simulink model "winter_simulink_with_PC_generator_control_EKF"  (R2022a)
settings: Solver=FixedStepAuto  StartTime=0  StopTime=50  FixedStep=simulation.time_step_H
values from neighbouring files (symbols this model uses):
  B_eq = param{6}    [measurement_2states.m]    (also in measurement_2states_3mes.m; measurement_3measure.m)
  rho = param{2}    [measurement_3measure.m]
undefined symbols (not defined in the file or in its folder): blade, Gc, gearbox, generator, generator_kd, generator_ki, generator_kp, generator_tau_d1, I_eq, IMM, lambda_vector, lookup_cP, omega_R, omega_rated, omega_rated_GE, pitch_range, pitch_vector, R_TG, rotor, simulation, T_R0, wind
settings Model: Creator=Niccolò  LastModifiedBy=Niccolò
settings SolverCC: ZeroCrossAlgorithm=Adaptive
settings DebuggingCC: IgnoredZcDiagnostic=none

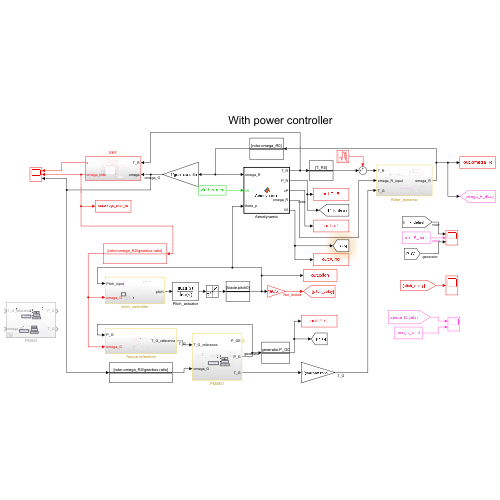
[thumbnail: Simulink's stored preview of the top-level diagram]
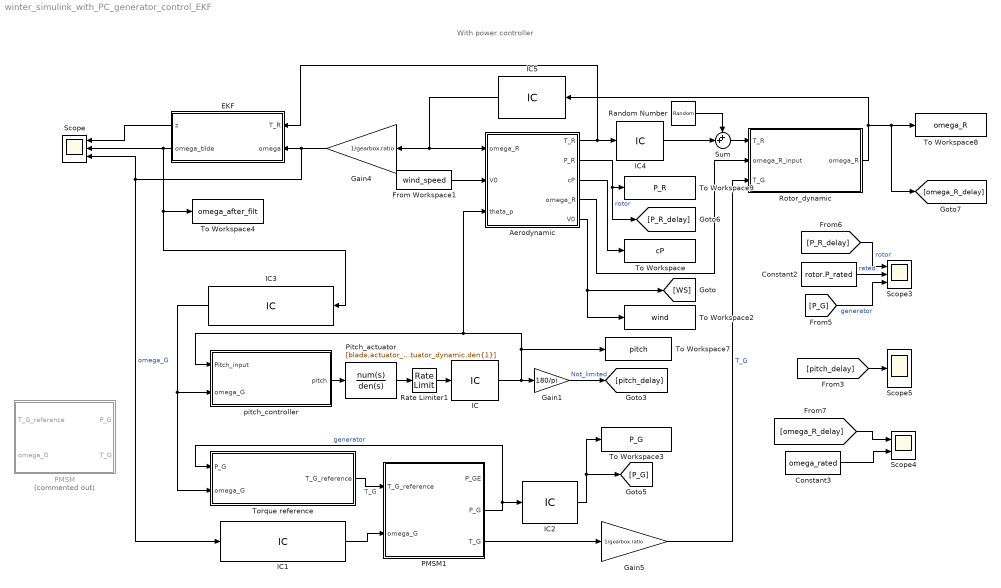
== system winter_simulink_with_PC_generator_control_EKF ==
  note: With power controller
  Aerodynamic : MATLAB Function  TreatAsAtomicUnit=on
  Constant2 : Constant  Value=rotor.P_rated
  Constant3 : Constant  Value=omega_rated
  EKF : Subsystem
  From Workspace1 : FromWorkspace  VariableName=wind_speed  SampleTime=1/wind.sample_f
  Gain1 : Gain  Gain=180/pi  SampleTime=simulation.time_step_H
  Gain4 : Gain  Gain=1/gearbox.ratio
  Gain5 : Gain  Gain=1/gearbox.ratio
  IC : InitialCondition  Value=blade.pitch0
  IC1 : InitialCondition  Value=rotor.omega_R0/gearbox.ratio
  IC2 : InitialCondition  Value=generator.P_G0
  IC3 : InitialCondition  Value=rotor.omega_R0/gearbox.ratio
  IC4 : InitialCondition  Value=T_R0
  IC5 : InitialCondition  Value=rotor.omega_R0
  PMSM : Subsystem  Commented=on
  PMSM1 : Subsystem
  Pitch_actuator : TransferFcn  Numerator=[blade.actuator_dynamic.num{1}]  Denominator=[blade.actuator_dynamic.den{1}]
  Random Number : RandomNumber  Variance=IMM.Q  SampleTime=simulation.time_step_H
  Rate Limiter1 : RateLimiter  RisingSlewLimit=blade.pitch_rate  FallingSlewLimit=-blade.pitch_rate  SampleTimeMode=inherited
  Rotor_dynamic : Subsystem
  Scope : Scope  NumInputPorts=3
  Scope3 : Scope  NumInputPorts=3
  Scope4 : Scope  NumInputPorts=2
  Scope5 : Scope
  Sum : Sum  Inputs=++|
  To Workspace : ToWorkspace  VariableName=cP  SaveFormat=Timeseries  SampleTime=-1
  To Workspace2 : ToWorkspace  VariableName=wind  SaveFormat=Timeseries  SampleTime=-1
  To Workspace3 : ToWorkspace  VariableName=P_G  SaveFormat=Timeseries  SampleTime=-1
  To Workspace4 : ToWorkspace  VariableName=omega_after_filt  SaveFormat=Timeseries  SampleTime=-1
  To Workspace7 : ToWorkspace  VariableName=pitch  SaveFormat=Timeseries  SampleTime=-1
  To Workspace8 : ToWorkspace  VariableName=omega_R  SaveFormat=Timeseries  SampleTime=-1
  To Workspace9 : ToWorkspace  VariableName=P_R  SaveFormat=Timeseries  SampleTime=-1
  Torque reference : Subsystem
  pitch_controller : Subsystem
  wires:
  From Workspace1/1 -> Aerodynamic/2("V0 ")
  Aerodynamic/2(P_R) -> [P_R_delay], To Workspace9/1  "rotor"
  [pitch_delay] -> Scope5/1
  Gain4/1 -> EKF/2(omega), IC1/1, Scope/3  "omega_G"
  Rate Limiter1/1 -> IC/1
  [P_R_delay] -> Scope3/1  "rotor"
  Constant3/1 -> Scope4/2
  Constant2/1 -> Scope3/2  "rated"
  [omega_R_delay] -> Scope4/1
  Gain1/1 -> [pitch_delay]  "Not_limited"
  Aerodynamic/1(T_R) -> EKF/1(T_R), IC4/1
  [P_G] -> Scope3/3  "generator"
  pitch_controller/1(pitch) -> Pitch_actuator/1
  Pitch_actuator/1 -> Rate Limiter1/1
  Gain5/1 -> Rotor_dynamic/3(T_G)  "T_G"
  IC/1 -> To Workspace7/1, Aerodynamic/3(theta_p), pitch_controller/1(Pitch_input), Gain1/1
  IC3/1 -> pitch_controller/2(omega_G), Torque reference/2(omega_G)
  IC2/1 -> To Workspace3/1, [P_G]
  IC4/1 -> Sum/2
  Rotor_dynamic/1(omega_R) -> IC5/1, [omega_R_delay], To Workspace8/1
  IC5/1 -> Aerodynamic/1("omega_R "), Gain4/1
  Aerodynamic/3(cP) -> To Workspace/1
  EKF/2(omega_tilde) -> To Workspace4/1, IC3/1, Scope/2
  Aerodynamic/4(omega_R) -> Rotor_dynamic/2(omega_R_input)
  Aerodynamic/5(V0) -> To Workspace2/1, [WS]
  PMSM1/2(P_G) -> Torque reference/1(P_G), IC2/1  "generator"
  IC1/1 -> PMSM1/2(omega_G)
  Torque reference/1(T_G_reference) -> PMSM1/1(T_G_reference)  "T_G"
  PMSM1/3(T_G) -> Gain5/1
  EKF/1(z) -> Scope/1
  Sum/1 -> Rotor_dynamic/1(T_R)
  Random Number/1 -> Sum/1

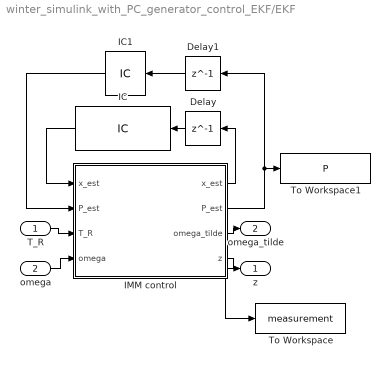
== system winter_simulink_with_PC_generator_control_EKF/EKF ==
  T_R : Inport
  omega : Inport  Port=2
  Delay : Delay  DelayLength=1
  Delay1 : Delay  DelayLength=1
  IC : InitialCondition  Value=rotor.omega_R0
  IC1 : InitialCondition  Value=1e2
  IMM control : MATLAB Function  TreatAsAtomicUnit=on
  To Workspace : ToWorkspace  VariableName=measurement  SaveFormat=Timeseries  SampleTime=-1
  To Workspace1 : ToWorkspace  VariableName=P  SaveFormat=Timeseries  SampleTime=-1
  z : Outport
  omega_tilde : Outport  Port=2
  wires:
  IMM control/3(omega_tilde) -> omega_tilde/1
  Delay1/1 -> IC1/1
  IMM control/1(x_est) -> Delay/1
  Delay/1 -> IC/1
  IMM control/2(P_est) -> Delay1/1, To Workspace1/1
  T_R/1 -> IMM control/3(T_R)
  omega/1 -> IMM control/4(omega)
  IC1/1 -> IMM control/2("P_est ")
  IC/1 -> IMM control/1("x_est ")
  IMM control/4(z) -> To Workspace/1, z/1

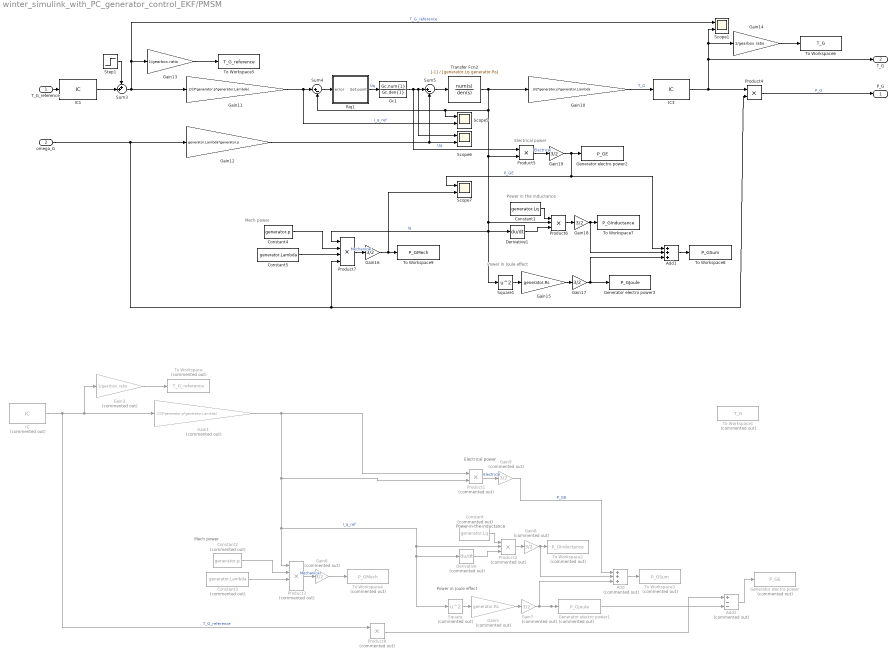
== system winter_simulink_with_PC_generator_control_EKF/PMSM ==
  note: Power in Joule effect
  note: Power in the inductance
  note: Electrical power
  note: Mech power
  note: Power in the inductance
  note: Electrical power
  note: Mech power
  note: Power in Joule effect
  T_G_reference : Inport
  omega_G : Inport  Port=2
  Add : Sum  Commented=on  Inputs=3
  Add1 : Sum  Inputs=3
  Add2 : Sum  Commented=on  Inputs=+--
  Constant : Constant  Commented=on  Value=generator.Lq
  Constant1 : Constant  Value=generator.Lq
  Constant2 : Constant  Commented=on  Value=generator.p
  Constant3 : Constant  Commented=on  Value=generator.Lambda
  Constant4 : Constant  Value=generator.p
  Constant5 : Constant  Value=generator.Lambda
  Derivative : Derivative  Commented=on
  Derivative1 : Derivative
  Gain1 : Gain  Commented=on  Gain=2/(3*generator.p*generator.Lambda)
  Gain10 : Gain  Gain=3/2*generator.p*generator.Lambda
  Gain11 : Gain  Gain=2/(3*generator.p*generator.Lambda)
  Gain12 : Gain  Gain=generator.Lambda*generator.p
  Gain13 : Gain  Gain=1/gearbox.ratio
  Gain14 : Gain  Gain=1/gearbox.ratio
  Gain15 : Gain  Gain=generator.Rs
  Gain{16..19} (4 alike) : Gain  Gain=3/2
  Gain3 : Gain  Commented=on  Gain=1/gearbox.ratio
  Gain5 : Gain  Commented=on  Gain=generator.Rs
  Gain{6..9} (4 alike) : Gain  Commented=on  Gain=3/2
  Gc1 : TransferFcn  Numerator=Gc.num{1}  Denominator=Gc.den{1}
  Generator electro power : ToWorkspace  Commented=on  VariableName=P_GE  SaveFormat=Timeseries  SampleTime=-1
  Generator electro power1 : ToWorkspace  Commented=on  VariableName=P_GJoule  SaveFormat=Timeseries  SampleTime=-1
  Generator electro power2 : ToWorkspace  VariableName=P_GE  SaveFormat=Timeseries  SampleTime=-1
  Generator electro power3 : ToWorkspace  VariableName=P_GJoule  SaveFormat=Timeseries  SampleTime=-1
  IC : InitialCondition  Commented=on  Value=generator.T_G0
  IC1 : InitialCondition  Value=generator.T_G0
  IC3 : InitialCondition  Value=generator.T_G0
  Product1 : Product  Commented=on
  Product2 : Product  Commented=on  Inputs=3
  Product3 : Product  Commented=on  Inputs=4
  Product4 : Product
  Product5 : Product
  Product6 : Product  Inputs=3
  Product7 : Product  Inputs=4
  Product8 : Product  Commented=on
  Riq1 : Subsystem
  Scope{1,5..7} (4 alike) : Scope  NumInputPorts=2
  Square : Math  Commented=on  Operator=square
  Square1 : Math  Operator=square
  Step1 : Step  Time=0.5  SampleTime=0
  Sum3 : Sum  Inputs=++|
  Sum4 : Sum  Inputs=|+-
  Sum5 : Sum  Inputs=|+-
  To Workspace : ToWorkspace  Commented=on  VariableName=T_G_reference  SaveFormat=Timeseries  SampleTime=-1
  To Workspace1 : ToWorkspace  Commented=on  VariableName=T_G  SaveFormat=Timeseries  SampleTime=-1
  To Workspace2 : ToWorkspace  Commented=on  VariableName=P_GInductance  SaveFormat=Timeseries  SampleTime=-1
  To Workspace3 : ToWorkspace  Commented=on  VariableName=P_GSum  SaveFormat=Timeseries  SampleTime=-1
  To Workspace4 : ToWorkspace  Commented=on  VariableName=P_GMech  SaveFormat=Timeseries  SampleTime=-1
  To Workspace5 : ToWorkspace  VariableName=T_G_reference  SaveFormat=Timeseries  SampleTime=-1
  To Workspace6 : ToWorkspace  VariableName=T_G  SaveFormat=Timeseries  SampleTime=-1
  To Workspace7 : ToWorkspace  VariableName=P_GInductance  SaveFormat=Timeseries  SampleTime=-1
  To Workspace8 : ToWorkspace  VariableName=P_GSum  SaveFormat=Timeseries  SampleTime=-1
  To Workspace9 : ToWorkspace  VariableName=P_GMech  SaveFormat=Timeseries  SampleTime=-1
  Transfer Fcn2 : TransferFcn  Numerator=[-1]  Denominator=[generator.Lq generator.Rs]
  P_G : Outport
  T_G : Outport  Port=2
  wires:
  Gain1/1 -> Product1/1, Square/1, Derivative/1, Product2/2, Product3/1, Product1/2  "I_q_ref"
  IC/1 -> Product8/1, Gain1/1, Gain3/1  "T_G_reference"
  Gain3/1 -> To Workspace/1
  Gain5/1 -> Gain7/1
  Square/1 -> Gain5/1
  Derivative/1 -> Product2/3
  Constant/1 -> Product2/1
  Product2/1 -> Gain8/1
  Add/1 -> To Workspace3/1
  Constant2/1 -> Product3/2
  Constant3/1 -> Product3/3
  Product3/1 -> Gain6/1  "Mechanical"
  Product1/1 -> Gain9/1  "Electrical"
  Gain6/1 -> To Workspace4/1
  Gain7/1 -> Add2/3, Generator electro power1/1, Add/3
  Gain8/1 -> Add/2, To Workspace2/1
  Gain9/1 -> Add/1  "P_GE"
  IC1/1 -> Sum3/2
  Product4/1 -> P_G/1  "P_G"
  Gain14/1 -> To Workspace6/1
  Gain19/1 -> Add1/1, Scope7/1, Generator electro power2/1  "P_GE"
  IC3/1 -> Product4/1, T_G/1, Scope1/2, Gain14/1
  Add1/1 -> To Workspace8/1
  Gain12/1 -> Scope6/2, Sum5/2
  Gain16/1 -> Scope7/2, To Workspace9/1
  Constant4/1 -> Product7/2
  omega_G/1 -> Product4/2, Product7/4, Gain12/1
  Square1/1 -> Gain15/1
  Constant5/1 -> Product7/3
  Product7/1 -> Gain16/1  "Mechanical"
  Derivative1/1 -> Product6/3
  Gain15/1 -> Gain17/1
  Constant1/1 -> Product6/1
  Product5/1 -> Gain19/1  "Electrical"
  Product6/1 -> Gain18/1
  Riq1/1(Set point) -> Gc1/1  "Uq"
  Gain11/1 -> Scope5/2, Sum4/1  "I_q_ref"
  Sum4/1 -> Riq1/1(error)
  Gain13/1 -> To Workspace5/1
  Step1/1 -> Sum3/1
  Gain10/1 -> IC3/1  "T_G"
  Sum3/1 -> Gain11/1, Scope1/1, Gain13/1  "T_G_reference"
  Transfer Fcn2/1 -> Gain10/1, Scope5/1, Sum4/2, Product5/2, Product7/1, Square1/1, Derivative1/1, Product6/2  "Iq"
  Sum5/1 -> Transfer Fcn2/1
  Gain18/1 -> To Workspace7/1, Add1/2
  Gain17/1 -> Generator electro power3/1, Add1/3
  Product8/1 -> Add2/1
  Add2/1 -> Generator electro power/1
  T_G_reference/1 -> IC1/1
  Gc1/1 -> Product5/1, Scope6/1, Sum5/1  "Uq"

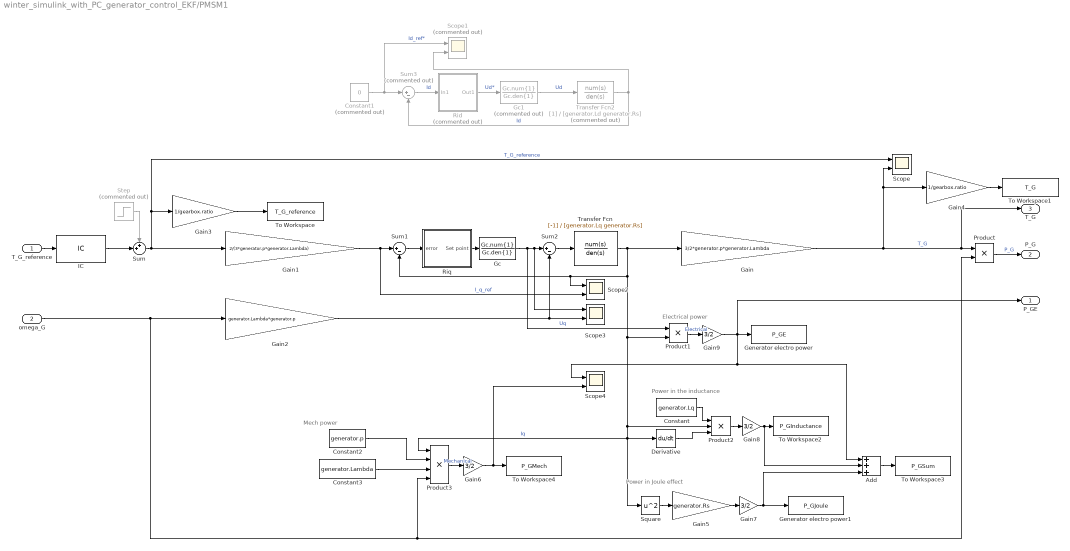
== system winter_simulink_with_PC_generator_control_EKF/PMSM1 ==
  note: Power in Joule effect
  note: Power in the inductance
  note: Electrical power
  note: Mech power
  T_G_reference : Inport
  omega_G : Inport  Port=2
  Add : Sum  Inputs=3
  Constant : Constant  Value=generator.Lq
  Constant1 : Constant  Commented=on  Value=0
  Constant2 : Constant  Value=generator.p
  Constant3 : Constant  Value=generator.Lambda
  Derivative : Derivative
  Gain : Gain  Gain=3/2*generator.p*generator.Lambda
  Gain1 : Gain  Gain=2/(3*generator.p*generator.Lambda)
  Gain2 : Gain  Gain=generator.Lambda*generator.p
  Gain3 : Gain  Gain=1/gearbox.ratio
  Gain4 : Gain  Gain=1/gearbox.ratio
  Gain5 : Gain  Gain=generator.Rs
  Gain{6..9} (4 alike) : Gain  Gain=3/2
  Gc : TransferFcn  Numerator=Gc.num{1}  Denominator=Gc.den{1}
  Gc1 : TransferFcn  Commented=on  Numerator=Gc.num{1}  Denominator=Gc.den{1}
  Generator electro power : ToWorkspace  VariableName=P_GE  SaveFormat=Timeseries  SampleTime=-1
  Generator electro power1 : ToWorkspace  VariableName=P_GJoule  SaveFormat=Timeseries  SampleTime=-1
  IC : InitialCondition  Value=generator.T_G0
  Product : Product
  Product1 : Product
  Product2 : Product  Inputs=3
  Product3 : Product  Inputs=4
  Rid : Subsystem  Commented=on
  Riq : Subsystem
  Scope{,2..4} (4 alike) : Scope  NumInputPorts=2
  Scope1 : Scope  Commented=on  NumInputPorts=2
  Square : Math  Operator=square
  Step : Step  Commented=on  Time=0.5  SampleTime=0
  Sum : Sum  Inputs=++|
  Sum1 : Sum  Inputs=|+-
  Sum2 : Sum  Inputs=|+-
  Sum3 : Sum  Commented=on  Inputs=|+-
  To Workspace : ToWorkspace  VariableName=T_G_reference  SaveFormat=Timeseries  SampleTime=-1
  To Workspace1 : ToWorkspace  VariableName=T_G  SaveFormat=Timeseries  SampleTime=-1
  To Workspace2 : ToWorkspace  VariableName=P_GInductance  SaveFormat=Timeseries  SampleTime=-1
  To Workspace3 : ToWorkspace  VariableName=P_GSum  SaveFormat=Timeseries  SampleTime=-1
  To Workspace4 : ToWorkspace  VariableName=P_GMech  SaveFormat=Timeseries  SampleTime=-1
  Transfer Fcn : TransferFcn  Numerator=[-1]  Denominator=[generator.Lq generator.Rs]
  Transfer Fcn2 : TransferFcn  Commented=on  Denominator=[generator.Ld generator.Rs]
  P_GE : Outport
  P_G : Outport  Port=2
  T_G : Outport  Port=3
  wires:
  Gc/1 -> Product1/1, Scope3/1, Sum2/1  "Uq"
  Gain/1 -> T_G/1, Product/1, Gain4/1, Scope/2  "T_G"
  Riq/1(Set point) -> Gc/1
  Sum1/1 -> Riq/1(error)
  Transfer Fcn/1 -> Gain/1, Scope2/1, Sum1/2, Product1/2, Product3/1, Square/1, Derivative/1, Product2/2  "Iq"
  Product/1 -> P_G/1  "P_G"
  Gain1/1 -> Scope2/2, Sum1/1  "I_q_ref"
  Sum/1 -> Gain1/1, Scope/1, Gain3/1  "T_G_reference"
  T_G_reference/1 -> IC/1
  Step/1 -> Sum/1
  Sum2/1 -> Transfer Fcn/1
  Gain3/1 -> To Workspace/1
  IC/1 -> Sum/2
  Gain5/1 -> Gain7/1
  Square/1 -> Gain5/1
  Derivative/1 -> Product2/3
  Constant/1 -> Product2/1
  Product2/1 -> Gain8/1
  Gc1/1 -> Transfer Fcn2/1  "Ud"
  Rid/1(Out1) -> Gc1/1  "Ud*"
  Transfer Fcn2/1 -> Sum3/2, Scope1/2  "Id"
  Constant1/1 -> Scope1/1, Sum3/1  "Id_ref*"
  Sum3/1 -> Rid/1(In1)  "Id"
  Add/1 -> To Workspace3/1
  Constant2/1 -> Product3/2
  Constant3/1 -> Product3/3
  Product3/1 -> Gain6/1  "Mechanical"
  Product1/1 -> Gain9/1  "Electrical"
  Gain2/1 -> Scope3/2, Sum2/2
  omega_G/1 -> Product/2, Product3/4, Gain2/1
  Gain6/1 -> Scope4/2, To Workspace4/1
  Gain7/1 -> Generator electro power1/1, Add/3
  Gain8/1 -> To Workspace2/1, Add/2
  Gain9/1 -> P_GE/1, Generator electro power/1, Add/1, Scope4/1
  Gain4/1 -> To Workspace1/1

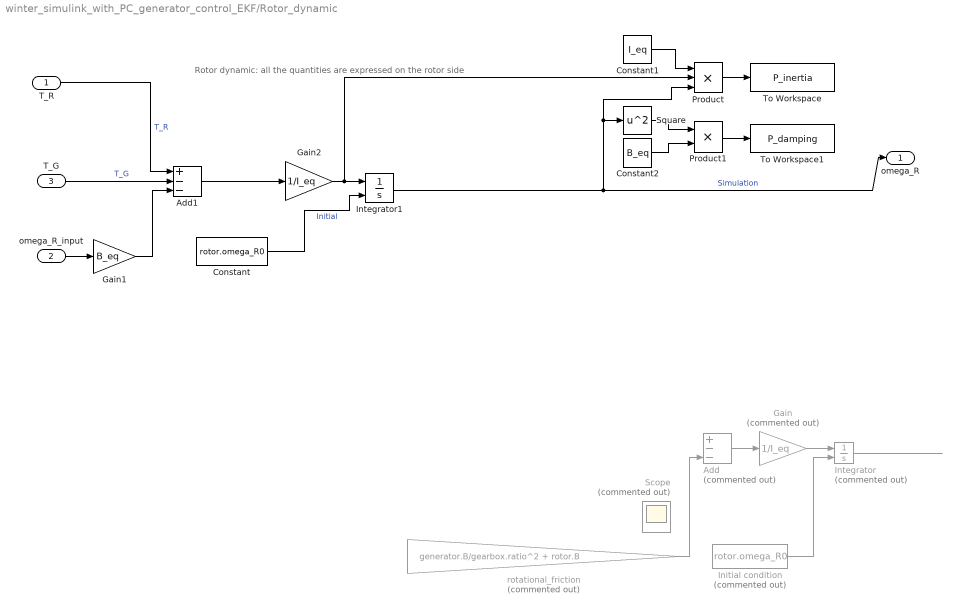
== system winter_simulink_with_PC_generator_control_EKF/Rotor_dynamic ==
  note: Rotor dynamic: all the quantities are expressed on the rotor side
  T_R : Inport
  omega_R_input : Inport  Port=2
  T_G : Inport  Port=3
  Add : Sum  Commented=on  Inputs=+--
  Add1 : Sum  Inputs=+--
  Constant : Constant  Value=rotor.omega_R0
  Constant1 : Constant  Value=I_eq
  Constant2 : Constant  Value=B_eq
  Gain : Gain  Commented=on  Gain=1/I_eq
  Gain1 : Gain  Gain=B_eq
  Gain2 : Gain  Gain=1/I_eq
  Initial condition : Constant  Commented=on  Value=rotor.omega_R0
  Integrator : Integrator  Commented=on  InitialConditionSource=external  InitialCondition=omega_R
  Integrator1 : Integrator  InitialConditionSource=external
  Product : Product  Inputs=3
  Product1 : Product
  Scope : Scope  Commented=on  NumInputPorts=2
  Square : Math  Operator=square
  To Workspace : ToWorkspace  VariableName=P_inertia  SaveFormat=Timeseries  SampleTime=-1
  To Workspace1 : ToWorkspace  VariableName=P_damping  SaveFormat=Timeseries  SampleTime=-1
  rotational_friction : Gain  Commented=on  Gain=generator.B/gearbox.ratio^2 + rotor.B
  omega_R : Outport
  wires:
  Integrator/1 -> ?
  Initial condition/1 -> Integrator/2
  Gain/1 -> Integrator/1
  Add/1 -> Gain/1
  rotational_friction/1 -> Add/3
  ? -> Add/1, Scope/1
  ? -> Add/2, Scope/2
  Gain2/1 -> Integrator1/1, Product/2
  omega_R_input/1 -> Gain1/1
  Gain1/1 -> Add1/3
  Add1/1 -> Gain2/1
  Constant2/1 -> Product1/2
  Square/1 -> Product1/1
  T_R/1 -> Add1/1  "T_R"
  Constant1/1 -> Product/1
  Product1/1 -> To Workspace1/1
  Integrator1/1 -> Product/3, Square/1, omega_R/1  "Simulation"
  Product/1 -> To Workspace/1
  T_G/1 -> Add1/2  "T_G"
  Constant/1 -> Integrator1/2  "Initial"

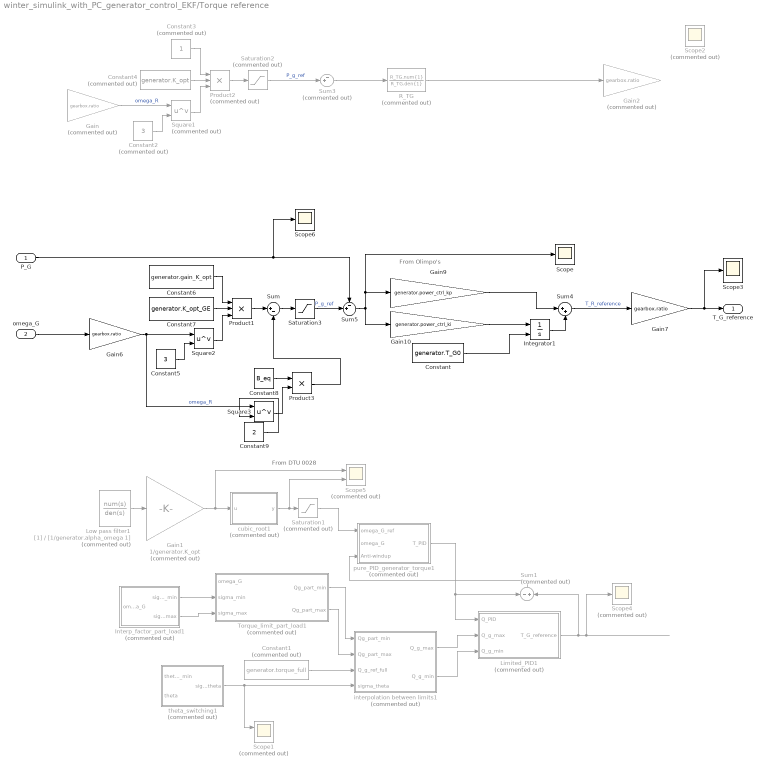
== system winter_simulink_with_PC_generator_control_EKF/Torque reference ==
  note: From DTU 0028
  note: From Olimpo's
  P_G : Inport
  omega_G : Inport  Port=2
  Constant : Constant  Value=generator.T_G0
  Constant1 : Constant  Commented=on  Value=generator.torque_full
  Constant2 : Constant  Commented=on  Value=3
  Constant3 : Constant  Commented=on
  Constant4 : Constant  Commented=on  Value=generator.K_opt
  Constant5 : Constant  Value=3
  Constant6 : Constant  Value=generator.gain_K_opt
  Constant7 : Constant  Value=generator.K_opt_GE
  Constant8 : Constant  Value=B_eq
  Constant9 : Constant  Value=2
  Gain : Gain  Commented=on  Gain=gearbox.ratio
  Gain1 : Gain  Commented=on  Gain=1/generator.K_opt
  Gain10 : Gain  Gain=generator.power_ctrl_ki
  Gain2 : Gain  Commented=on  Gain=gearbox.ratio
  Gain6 : Gain  Gain=gearbox.ratio
  Gain7 : Gain  Gain=gearbox.ratio
  Gain9 : Gain  Gain=generator.power_ctrl_kp
  Integrator1 : Integrator  InitialConditionSource=external
  Interp_factor_part_load1 : Subsystem  Commented=on
  Limited_PID1 : Subsystem  Commented=on
  Low pass filter1 : TransferFcn  Commented=on  Denominator=[1/generator.alpha_omega 1]
  Product1 : Product  Inputs=3
  Product2 : Product  Commented=on  Inputs=3
  Product3 : Product
  R_TG : TransferFcn  Commented=on  Numerator=R_TG.num{1}  Denominator=R_TG.den{1}
  Saturation1 : Saturate  Commented=on  UpperLimit=generator.omega_rated  LowerLimit=0
  Saturation2 : Saturate  Commented=on  UpperLimit=rotor.P_rated  LowerLimit=0
  Saturation3 : Saturate  UpperLimit=generator.P_rated  LowerLimit=0
  Scope : Scope
  Scope1 : Scope  Commented=on  NumInputPorts=2
  Scope2 : Scope  Commented=on
  Scope3 : Scope
  Scope4 : Scope  Commented=on
  Scope5 : Scope  Commented=on  NumInputPorts=2
  Scope6 : Scope
  Square1 : Math  Commented=on  Operator=pow
  Square2 : Math  Operator=pow
  Square3 : Math  Operator=pow
  Sum : Sum  Inputs=|+-
  Sum1 : Sum  Commented=on  Inputs=-|+
  Sum3 : Sum  Commented=on  Inputs=-+|
  Sum4 : Sum  Inputs=|++
  Sum5 : Sum  Inputs=-+|
  Torque_limit_part_load1 : Subsystem  Commented=on
  cubic_root1 : MATLAB Function  Commented=on  TreatAsAtomicUnit=on
  interpolation between limits1 : MATLAB Function  Commented=on  TreatAsAtomicUnit=on
  pure_PID_generator_torque1 : Subsystem  Commented=on
  theta_switching1 : Subsystem  Commented=on
  T_G_reference : Outport
  wires:
  theta_switching1/1(sigma_theta) -> Scope1/1, interpolation between limits1/4(sigma_theta)
  Limited_PID1/1(T_G_reference) -> Sum1/2, Scope4/1
  Interp_factor_part_load1/2(sigma_max) -> Torque_limit_part_load1/3(sigma_max)
  ? -> theta_switching1/1(theta_min)
  ? -> theta_switching1/2(theta)
  pure_PID_generator_torque1/1(T_PID) -> Limited_PID1/1(Q_PID), Sum1/1
  Constant1/1 -> interpolation between limits1/3(Q_g_ref_full)
  cubic_root1/1(y) -> Scope5/2, Saturation1/1
  Interp_factor_part_load1/1(sigma_min) -> Torque_limit_part_load1/2(sigma_min)
  ? -> Torque_limit_part_load1/1(omega_G), pure_PID_generator_torque1/2(omega_G), Interp_factor_part_load1/1(omega_G), Scope1/2
  Gain1/1 -> Scope5/1, cubic_root1/1(u)
  Sum1/1 -> pure_PID_generator_torque1/3(Anti-windup)
  Torque_limit_part_load1/2(Qg_part_max) -> interpolation between limits1/2(Qg_part_max)
  Saturation1/1 -> pure_PID_generator_torque1/1(omega_G_ref)
  Torque_limit_part_load1/1(Qg_part_min) -> interpolation between limits1/1(Qg_part_min)
  Low pass filter1/1 -> Gain1/1
  interpolation between limits1/2(Q_g_min) -> Limited_PID1/3(Q_g_min)
  interpolation between limits1/1(Q_g_max) -> Limited_PID1/2(Q_g_max)
  Square2/1 -> Product1/3
  Gain9/1 -> Sum4/1
  omega_G/1 -> Gain6/1
  Gain10/1 -> Integrator1/1
  Constant/1 -> Integrator1/2
  Sum4/1 -> Gain7/1  "T_R_reference"
  Constant6/1 -> Product1/1
  Constant5/1 -> Square2/2
  Saturation3/1 -> Sum5/2  "P_g_ref"
  Constant7/1 -> Product1/2
  Integrator1/1 -> Sum4/2
  Sum5/1 -> Scope/1, Gain9/1, Gain10/1
  R_TG/1 -> Gain2/1
  Square1/1 -> Product2/3
  Sum3/1 -> R_TG/1
  Constant2/1 -> Square1/2
  ? -> Sum3/1
  Constant3/1 -> Product2/1
  Gain/1 -> Square1/1  "omega_R"
  Product2/1 -> Saturation2/1
  Saturation2/1 -> Sum3/2  "P_g_ref"
  ? -> Gain/1
  Constant4/1 -> Product2/2
  P_G/1 -> Scope6/1, Sum5/1
  Gain7/1 -> T_G_reference/1, Scope3/1
  Product1/1 -> Sum/1
  Sum/1 -> Saturation3/1
  Constant9/1 -> Square3/2
  Gain6/1 -> Square3/1, Square2/1  "omega_R"
  Square3/1 -> Product3/2
  Constant8/1 -> Product3/1
  Product3/1 -> Sum/2

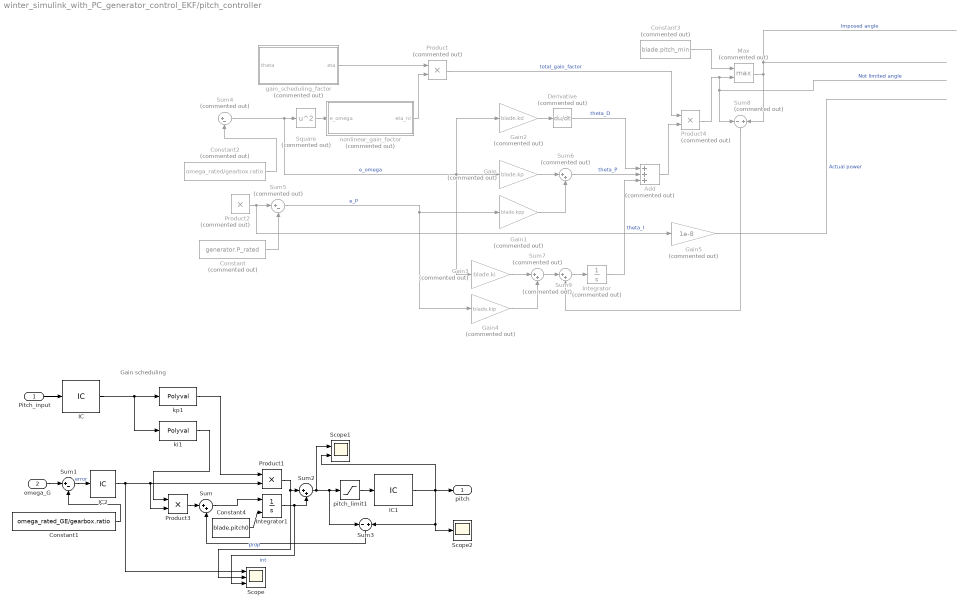
== system winter_simulink_with_PC_generator_control_EKF/pitch_controller ==
  note: Gain scheduling
  Pitch_input : Inport
  omega_G : Inport  Port=2
  Add : Sum  Commented=on  Inputs=+++
  Constant : Constant  Commented=on  Value=generator.P_rated
  Constant1 : Constant  Value=omega_rated_GE/gearbox.ratio
  Constant2 : Constant  Commented=on  Value=omega_rated/gearbox.ratio
  Constant3 : Constant  Commented=on  Value=blade.pitch_min
  Constant4 : Constant  Value=blade.pitch0
  Derivative : Derivative  Commented=on
  Gain : Gain  Commented=on  Gain=blade.kp
  Gain1 : Gain  Commented=on  Gain=blade.kpp
  Gain2 : Gain  Commented=on  Gain=blade.kd
  Gain3 : Gain  Commented=on  Gain=blade.ki
  Gain4 : Gain  Commented=on  Gain=blade.kip
  Gain5 : Gain  Commented=on  Gain=1e-8
  IC : InitialCondition  Value=blade.pitch0
  IC1 : InitialCondition  Value=blade.pitch0
  IC2 : InitialCondition  Value=(rotor.omega_R0 - omega_rated)/gearbox.ratio
  Integrator : Integrator  Commented=on
  Integrator1 : Integrator  InitialConditionSource=external
  Max : MinMax  Commented=on  Function=max  Inputs=2
  Product : Product  Commented=on
  Product1 : Product
  Product2 : Product  Commented=on
  Product3 : Product
  Product4 : Product  Commented=on
  Scope : Scope  NumInputPorts=3
  Scope1 : Scope  NumInputPorts=2
  Scope2 : Scope
  Square : Math  Commented=on  Operator=square
  Sum : Sum  Inputs=|++
  Sum1 : Sum  Inputs=|+-
  Sum2 : Sum  Inputs=|++
  Sum3 : Sum  Inputs=-|+
  Sum4 : Sum  Commented=on  Inputs=|+-
  Sum5 : Sum  Commented=on  Inputs=|+-
  Sum6 : Sum  Commented=on  Inputs=|++
  Sum7 : Sum  Commented=on  Inputs=|++
  Sum8 : Sum  Commented=on  Inputs=-|+
  Sum9 : Sum  Commented=on  Inputs=|++
  gain_scheduling_factor : MATLAB Function  Commented=on  TreatAsAtomicUnit=on
  ki1 : Polyval  Coefs=blade.ki_schedule
  kp1 : Polyval  Coefs=blade.kp_schedule
  nonlinear_gain_factor : MATLAB Function  Commented=on  TreatAsAtomicUnit=on
  pitch_limit1 : Saturate  UpperLimit=pitch_range(2)  LowerLimit=0
  pitch : Outport
  wires:
  Sum/1 -> Integrator1/1
  Constant1/1 -> Sum1/2
  Product3/1 -> Sum/1
  omega_G/1 -> Sum1/1
  ki1/1 -> Product3/1
  kp1/1 -> Product1/1
  Sum1/1 -> IC2/1  "error"
  Product1/1 -> Scope/2, Sum2/1  "prop"
  Integrator1/1 -> Scope/3, Sum2/2  "int"
  ? -> ?  "Actual value"
  Sum8/1 -> Sum9/2
  Product4/1 -> Max/2, Sum8/1  "Not limited angle"
  Add/1 -> Product4/2
  Gain4/1 -> Sum7/2
  Product2/1 -> Gain5/1, Sum5/1
  Integrator/1 -> Add/3  "theta_I"
  ? -> Product2/2
  Derivative/1 -> Add/1  "theta_D"
  Product/1 -> Product4/1  "total_gain_factor"
  Sum6/1 -> Add/2  "theta_P"
  nonlinear_gain_factor/1(eta_nl) -> Product/2
  gain_scheduling_factor/1(eta) -> Product/1
  Gain/1 -> Sum6/1
  Max/1 -> Sum8/2  "Imposed angle"
  Sum5/1 -> Gain4/1, Gain1/1  "e_P"
  ? -> Sum4/1, Product2/1
  Constant2/1 -> Sum4/2
  Sum4/1 -> Gain3/1, Gain2/1, Gain/1, Square/1  "e_omega"
  Gain2/1 -> Derivative/1
  ? -> gain_scheduling_factor/1(theta)
  Gain5/1 -> ?  "Actual power"
  Constant/1 -> Sum5/2
  Constant3/1 -> Max/1
  Sum9/1 -> Integrator/1
  Gain1/1 -> Sum6/2
  Sum7/1 -> Sum9/1
  Square/1 -> nonlinear_gain_factor/1(e_omega)
  Gain3/1 -> Sum7/1
  Pitch_input/1 -> IC/1
  Sum2/1 -> pitch_limit1/1, Sum3/1, Scope1/1
  Sum3/1 -> Sum/2
  pitch_limit1/1 -> IC1/1
  IC/1 -> ki1/1, kp1/1
  IC1/1 -> Scope1/2, pitch/1, Scope2/1, Sum3/2
  IC2/1 -> Scope/1, Product3/2, Product1/2
  Constant4/1 -> Integrator1/2

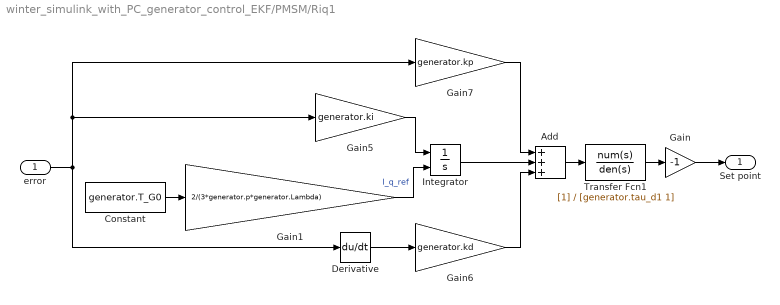
== system winter_simulink_with_PC_generator_control_EKF/PMSM/Riq1 ==
  error : Inport
  Add : Sum  Inputs=+++
  Constant : Constant  Value=generator.T_G0
  Derivative : Derivative
  Gain : Gain  Gain=-1
  Gain1 : Gain  Gain=2/(3*generator.p*generator.Lambda)
  Gain5 : Gain  Gain=generator.ki
  Gain6 : Gain  Gain=generator.kd
  Gain7 : Gain  Gain=generator.kp
  Integrator : Integrator  InitialConditionSource=external
  Transfer Fcn1 : TransferFcn  Denominator=[generator.tau_d1 1]
  Set point : Outport
  wires:
  Integrator/1 -> Add/2
  Constant/1 -> Gain1/1
  Gain7/1 -> Add/1
  Gain6/1 -> Add/3
  Derivative/1 -> Gain6/1
  error/1 -> Gain5/1, Gain7/1, Derivative/1
  Gain5/1 -> Integrator/1
  Gain1/1 -> Integrator/2  "I_q_ref"
  Gain/1 -> Set point/1
  Add/1 -> Transfer Fcn1/1
  Transfer Fcn1/1 -> Gain/1

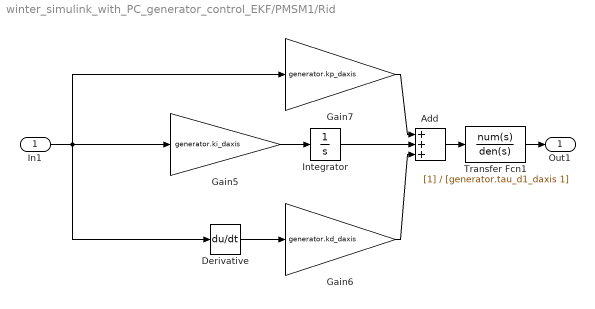
== system winter_simulink_with_PC_generator_control_EKF/PMSM1/Rid ==
  In1 : Inport
  Add : Sum  Inputs=+++
  Derivative : Derivative
  Gain5 : Gain  Gain=generator.ki_daxis
  Gain6 : Gain  Gain=generator.kd_daxis
  Gain7 : Gain  Gain=generator.kp_daxis
  Integrator : Integrator
  Transfer Fcn1 : TransferFcn  Denominator=[generator.tau_d1_daxis 1]
  Out1 : Outport
  wires:
  Integrator/1 -> Add/2
  Add/1 -> Transfer Fcn1/1
  Gain7/1 -> Add/1
  Gain6/1 -> Add/3
  Derivative/1 -> Gain6/1
  In1/1 -> Derivative/1, Gain7/1, Gain5/1
  Transfer Fcn1/1 -> Out1/1
  Gain5/1 -> Integrator/1

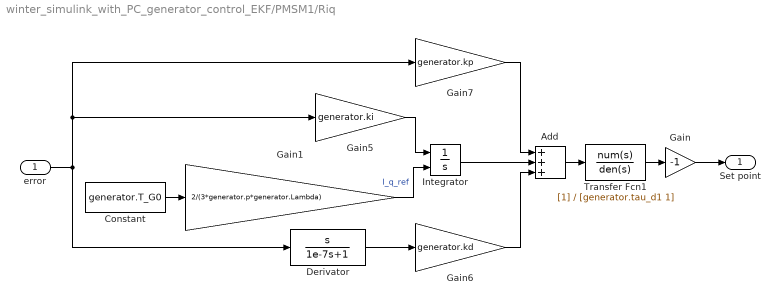
== system winter_simulink_with_PC_generator_control_EKF/PMSM1/Riq ==
  error : Inport
  Add : Sum  Inputs=+++
  Constant : Constant  Value=generator.T_G0
  Derivator : TransferFcn  Numerator=[1 0]  Denominator=[1e-7 1]
  Gain : Gain  Gain=-1
  Gain1 : Gain  Gain=2/(3*generator.p*generator.Lambda)
  Gain5 : Gain  Gain=generator.ki
  Gain6 : Gain  Gain=generator.kd
  Gain7 : Gain  Gain=generator.kp
  Integrator : Integrator  InitialConditionSource=external
  Transfer Fcn1 : TransferFcn  Denominator=[generator.tau_d1 1]
  Set point : Outport
  wires:
  Integrator/1 -> Add/2
  Add/1 -> Transfer Fcn1/1
  Constant/1 -> Gain1/1
  Gain7/1 -> Add/1
  Gain6/1 -> Add/3
  Derivator/1 -> Gain6/1
  error/1 -> Derivator/1, Gain5/1, Gain7/1
  Transfer Fcn1/1 -> Gain/1
  Gain5/1 -> Integrator/1
  Gain1/1 -> Integrator/2  "I_q_ref"
  Gain/1 -> Set point/1

== system winter_simulink_with_PC_generator_control_EKF/Torque reference/Interp_factor_part_load1 ==
  omega_G : Inport
  Scope : Scope  NumInputPorts=2
  sigma_function_speed : MATLAB Function  TreatAsAtomicUnit=on
  sigma_min : Outport
  sigma_max : Outport  Port=2
  wires:
  omega_G/1 -> sigma_function_speed/1(omega)
  sigma_function_speed/1(sigma_min) -> Scope/1, sigma_min/1  "min"
  sigma_function_speed/2(sigma_max) -> Scope/2, sigma_max/1  "max"

== system winter_simulink_with_PC_generator_control_EKF/Torque reference/Limited_PID1 ==
  Q_PID : Inport
  Q_g_max : Inport  Port=2
  Q_g_min : Inport  Port=3
  Max : MinMax  Function=max  Inputs=2
  Min : MinMax  Inputs=2
  torque_command : Scope  NumInputPorts=3
  T_G_reference : Outport
  wires:
  Min/1 -> Max/1
  Q_g_min/1 -> torque_command/3, Max/2  "Q g min"
  Q_g_max/1 -> torque_command/2, Min/2  "Q g max"
  Q_PID/1 -> torque_command/1, Min/1  "Q pid"
  Max/1 -> T_G_reference/1

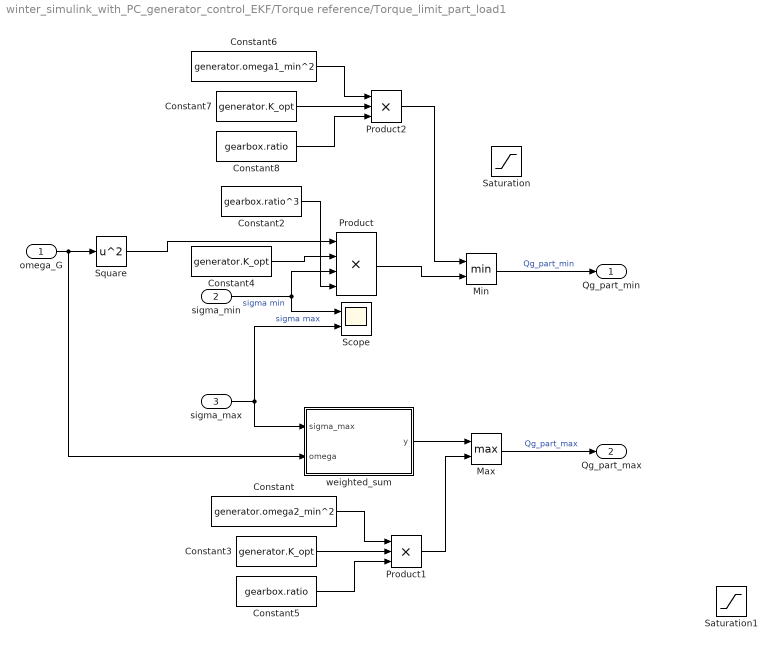
== system winter_simulink_with_PC_generator_control_EKF/Torque reference/Torque_limit_part_load1 ==
  omega_G : Inport
  sigma_min : Inport  Port=2
  sigma_max : Inport  Port=3
  Constant : Constant  Value=generator.omega2_min^2
  Constant2 : Constant  Value=gearbox.ratio^3
  Constant3 : Constant  Value=generator.K_opt
  Constant4 : Constant  Value=generator.K_opt
  Constant5 : Constant  Value=gearbox.ratio
  Constant6 : Constant  Value=generator.omega1_min^2
  Constant7 : Constant  Value=generator.K_opt
  Constant8 : Constant  Value=gearbox.ratio
  Max : MinMax  Function=max  Inputs=2
  Min : MinMax  Inputs=2
  Product : Product  Inputs=4
  Product1 : Product  Inputs=3
  Product2 : Product  Inputs=3
  Saturation : Saturate  UpperLimit=generator.K_opt*generator.omega2_max^2*gearbox.ratio  LowerLimit=-inf
  Saturation1 : Saturate  UpperLimit=inf  LowerLimit=generator.K_opt*generator.omega2_min^2*gearbox.ratio
  Scope : Scope  NumInputPorts=2
  Square : Math  Operator=square
  weighted_sum : MATLAB Function  TreatAsAtomicUnit=on
  Qg_part_min : Outport
  Qg_part_max : Outport  Port=2
  wires:
  weighted_sum/1(y) -> Max/1
  Constant4/1 -> Product/2
  Max/1 -> Qg_part_max/1  "Qg_part_max"
  Min/1 -> Qg_part_min/1  "Qg_part_min"
  sigma_min/1 -> Product/3, Scope/1  "sigma min"
  sigma_max/1 -> Scope/2, weighted_sum/1(sigma_max)  "sigma max"
  omega_G/1 -> weighted_sum/2(omega), Square/1
  Square/1 -> Product/1
  Constant2/1 -> Product/4
  Product1/1 -> Max/2
  Constant/1 -> Product1/1
  Constant3/1 -> Product1/2
  Constant5/1 -> Product1/3
  Constant7/1 -> Product2/2
  Product2/1 -> Min/1
  Constant8/1 -> Product2/3
  Constant6/1 -> Product2/1
  Product/1 -> Min/2

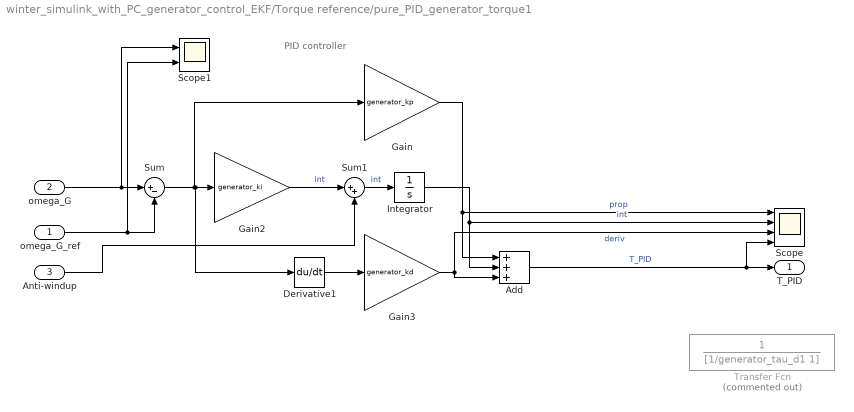
== system winter_simulink_with_PC_generator_control_EKF/Torque reference/pure_PID_generator_torque1 ==
  note: PID controller
  omega_G_ref : Inport
  omega_G : Inport  Port=2
  Anti-windup : Inport  Port=3
  Add : Sum  Inputs=+++
  Derivative1 : Derivative
  Gain : Gain  Gain=generator_kp
  Gain2 : Gain  Gain=generator_ki
  Gain3 : Gain  Gain=generator_kd
  Integrator : Integrator
  Scope : Scope  NumInputPorts=4
  Scope1 : Scope  NumInputPorts=2
  Sum : Sum  Inputs=|+-
  Sum1 : Sum  Inputs=|++
  Transfer Fcn : TransferFcn  Commented=on  Denominator=[1/generator_tau_d1 1]
  T_PID : Outport
  wires:
  omega_G/1 -> Scope1/1, Sum/1
  omega_G_ref/1 -> Scope1/2, Sum/2
  Derivative1/1 -> Gain3/1
  Sum/1 -> Gain2/1, Derivative1/1, Gain/1
  Gain3/1 -> Add/3, Scope/3  "deriv"
  Integrator/1 -> Scope/2, Add/2  "int"
  Gain/1 -> Scope/1, Add/1  "prop"
  Add/1 -> Scope/4, T_PID/1  "T_PID"
  Anti-windup/1 -> Sum1/2
  Sum1/1 -> Integrator/1  "int"
  Gain2/1 -> Sum1/1  "int"

== system winter_simulink_with_PC_generator_control_EKF/Torque reference/theta_switching1 ==
  theta_min : Inport
  theta : Inport  Port=2
  Add1 : Sum
  Constant5 : Constant  Value=blade.theta_f
  MATLAB Function1 : MATLAB Function  TreatAsAtomicUnit=on
  Saturation3 : Saturate  UpperLimit=1  LowerLimit=0
  Scope : Scope  NumInputPorts=3
  sigma_theta : Outport
  wires:
  theta/1 -> Scope/1, MATLAB Function1/1(theta)  "theta"
  Constant5/1 -> Add1/2
  Add1/1 -> Scope/3, MATLAB Function1/3(theta_max)  "theta_max"
  Saturation3/1 -> sigma_theta/1
  MATLAB Function1/1(sigma_theta) -> Saturation3/1
  theta_min/1 -> Scope/2, MATLAB Function1/2(theta_min), Add1/1  "theta_min"

== matlab function winter_simulink_with_PC_generator_control_EKF/pitch_controller/gain_scheduling_factor ==
  data: eta output; theta input; blade parameter
function eta = gain_scheduling_factor(theta, blade)

K1 = blade.K1;
K2 = blade.K2;

theta = theta*180/pi; % [deg]

eta = 1/(1+ theta/K1 + theta^2/K2);

== matlab function winter_simulink_with_PC_generator_control_EKF/Torque reference/theta_switching1/MATLAB Function1 ==
  data: theta input; sigma_theta output; theta_min input; theta_max input
function sigma_theta = fcn(theta, theta_min, theta_max)


sigma_theta = (theta - theta_min)/(theta_max - theta_min);

== matlab function winter_simulink_with_PC_generator_control_EKF/pitch_controller/nonlinear_gain_factor ==
  data: e_omega input; eta_nl output; blade parameter; generator parameter
function eta_nl = nonlinear_gain_factor(e_omega, blade, generator)

omega_rated = generator.omega_rated;
omega2 = omega_rated*blade.omega2omega0ratio;

eta_nl = 1 + e_omega^2/(omega2 - omega_rated)^2;

== matlab function winter_simulink_with_PC_generator_control_EKF/Torque reference/Interp_factor_part_load1/sigma_function_speed ==
  data: sigma_min output; omega input; sigma_max output; generator parameter
function [sigma_min, sigma_max] = sigma_fcn(omega, generator)

omega1_min = generator.omega1_min;
omega1_max = generator.omega1_max;
omega2_min = generator.omega2_min;
omega2_max = generator.omega2_max;

if generator.omega1_min == 0
  sigma_min = 1;
else
  sigma_min = sigma(omega1_min, omega2_min, omega);
end

sigma_max = sigma(omega1_max, omega2_max, omega);


function y = sigma(x0, x1, x)
  a = [2 -3*(x0 + x1) 6*x1*x0 (x0 - 3*x1)*x0^2]/(x0 - x1)^3;  % poly coeff.

  if x < x0
    y = 0;
  elseif x0 <= x && x <= x1
    y = polyval(a, x);  
  else 
    y = 1;
  end
end

end

== matlab function winter_simulink_with_PC_generator_control_EKF/Aerodynamic ==
  data: omega_R input; V0 input; T_R output; P_R output; rho parameter; theta_p input; lambda_vector parameter; pitch_vector parameter; lookup_cP parameter; cP output; rotor parameter; omega_R output; V0 output
function [T_R, P_R, cP, omega_R, V0] = Aerodynamic(omega_R, V0, rho, theta_p, lambda_vector, pitch_vector, lookup_cP, rotor) 

R = rotor.R;                  % rotor radius [m]

% retrive the cP from the look-up table
lambda = omega_R*R/V0;                                                
cP = interp2(lambda_vector, pitch_vector, lookup_cP, lambda, theta_p);

P_R = 0.5*rho*V0^3*pi*R^2*cP; % rotor power [W]
T_R = P_R/omega_R;            % rotor torque [Nm]

== matlab function winter_simulink_with_PC_generator_control_EKF/EKF/IMM control ==
  settings: updateMethod=DISCRETE  sampleTime=simulation.time_step_H
  data: x_est output; P_est output; x_est input size=[IMM.states_len]; P_est input size=[IMM.states_len, IMM.states_len]; T_R input; omega input; IMM parameter; I_eq parameter; omega_tilde output size=1; B_eq parameter; z output; generator parameter
function [x_est, P_est, omega_tilde, z] = gain_IMM(x_est, P_est, T_R, omega, IMM, I_eq, B_eq, generator)
  % x_est -> (states_len, n_models) items containing the state estimation
  % P_est -> (states_len, states_len, n_models) containing the covariance
  
  states_len = 1; % length of the states
  R = IMM.W;
  Q = IMM.Q;
  % Vector of parameters
  param = cell(5,1);
  param{1} = I_eq; % inertia
  param{2} = B_eq; % damping
  param{3} = generator.K_opt_GE;
  param{4} = R; % measure noise
  param{5} = Q; % process noise 
  x_real = [omega];
  omega_tilde = zeros(1);
  
  % Assamble the model cell
  model = cell(1, 1);

  model{1} = struct('K_opt', generator.K_opt_GE, 'x_est', x_est(1:states_len, 1), 'P_est', P_est(1:states_len,1:states_len));
  
  % Simulate the measurement
  z = measurement(x_real, param{5}) + my_mvnrnd([0], R, 1)'; % rotational speed measurement [rad/s]
  
  % Filtering
  model = filtering(model, z, T_R, param);
  
  % Estimation of the rotational speed
  omega_tilde = model{1}.x_est(1);

  x_est = model{1}.x_est;
  P_est = model{1}.P_est;

  end
  
  %   _____ _  _______ 
  %  | ____| |/ /  ___|
  %  |  _| | ' /| |_   
  %  | |___| . \|  _|  
  %  |_____|_|\_\_|    
                     
  function [model] = EKF(model, z, T_R, param, matrices)
    % y -> measurement of the rotational speed [rad/s]
    
    x_est = model.x_est;
    P_est = model.P_est;
    states_len = size(x_est, 2);
  
    F = matrices.F;
    H = matrices.H;
    Q = matrices.Q;
    R = matrices.R;
    G = matrices.G;
  
    % Prediction
    x_est = dynamic(x_est(1:states_len), T_R, param);
    P_est = F*P_est*F' + G*Q*G';
    states_len = size(x_est, 1); % number of states
  
    % Update
    [~, z_hat] = measurement(x_est, param{4}); % estimation of the measurement using the sensor's model
    Innovation = z - z_hat;
    S_Inno = H*P_est*H' + R;
    W = P_est*H'*inv(S_Inno); % kalman gain
    x_est = x_est + W*Innovation; % update state estimate
    P_est = (eye(states_len) - W*H)*P_est; % update covariance matrix
  
    model.x_est(1:states_len) = x_est(1:states_len);
    model.P_est(1:states_len, 1:states_len) = P_est(1:states_len, 1:states_len);
  end
  
  %   ____                              _      
  %  |  _ \ _   _ _ __   __ _ _ __ ___ (_) ___ 
  %  | | | | | | | '_ \ / _` | '_ ` _ \| |/ __|
  %  | |_| | |_| | | | | (_| | | | | | | | (__ 
  %  |____/ \__, |_| |_|\__,_|_| |_| |_|_|\___|
  %         |___/                              
  
  function x_new = dynamic(x_est, T_R, param)
  
    states_len = size(x_est, 1);
    I_eq = param{1}; % Inertia
    B_eq = param{2}; % Damping
    K_opt = param{3}; % Power coefficient
    x_new = zeros(states_len,1);
  
    x_new(1) = x_est(1) + 1/I_eq*(T_R - K_opt*x_est(1)^2);% - B_eq*x_est(1));
  end
  
  %   __  __                                                    _   
  %  |  \/  | ___  __ _ ___ _   _ _ __ ___ _ __ ___   ___ _ __ | |_ 
  %  | |\/| |/ _ \/ _` / __| | | | '__/ _ \ '_ ` _ \ / _ \ '_ \| __|
  %  | |  | |  __/ (_| \__ \ |_| | | |  __/ | | | | |  __/ | | | |_ 
  %  |_|  |_|\___|\__,_|___/\__,_|_|  \___|_| |_| |_|\___|_| |_|\__|
                                       
  function [z, z_hat] = measurement(x, R)
    % z_hat -> fake measuerement to be used in the KF
  
    z_hat = x(1); % rotational speed [rad/s]
    z = x(1); %+ mvnrnd([0], R)'; % rotational speed [rad/s]
  end
  
  %    ____                            _                         _     
  %   / ___|___  _ __ ___  _ __  _   _| |_ ___   _ __ ___   __ _| |_   
  %  | |   / _ \| '_ ` _ \| '_ \| | | | __/ _ \ | '_ ` _ \ / _` | __|  
  %  | |__| (_) | | | | | | |_) | |_| | ||  __/ | | | | | | (_| | |_ _ 
  %   \____\___/|_| |_| |_| .__/ \__,_|\__\___| |_| |_| |_|\__,_|\__(_)
  %                       |_|                                          
  
  function matrices = compute_matrices(x_est, param)
  
    I_eq = param{1}; % Inertia
    B_eq = param{2}; % Density
    K_opt = param{3}; % Power coefficient
  
    F = [-2*K_opt/I_eq*x_est(1)];%-B_eq/I_eq];
    H = [1];
    G = [1/I_eq];
  %   matrices = cell(4, 1);
    matrices = struct('F', F, 'H', H, 'G', G);
  end
  
  %   _____ _ _ _            _             
  %  |  ___(_) | |_ ___ _ __(_)_ __   __ _ 
  %  | |_  | | | __/ _ \ '__| | '_ \ / _` |
  %  |  _| | | | ||  __/ |  | | | | | (_| |
  %  |_|   |_|_|\__\___|_|  |_|_| |_|\__, |
  %                                  |___/ 
  
  function model = filtering(model, z, T_G, param)
    n_models = size(model, 1);
    states_len = size(model{1}.x_est, 2);
  
    param{3} = model{1}.K_opt;
    % compute the linearized matrices
    matrices = compute_matrices(model{1}.x_est(1:states_len), param);
    matrices.R = param{4};
    matrices.Q = param{5};

    [model{1}] = EKF(model{1}, z, T_G, param, matrices);

  end
  
  %                                       _ 
  %   _ __ _____   ___ __  _ __ _ __   __| |
  %  | '_ ` _ \ \ / / '_ \| '__| '_ \ / _` |
  %  | | | | | \ V /| | | | |  | | | | (_| |
  %  |_| |_| |_|\_/ |_| |_|_|  |_| |_|\__,_|
                                          
  function y = my_mvnrnd(mu, cov, n)
      % Cholesky decomposition
      L = chol(cov, 'lower');
  
      % Generate standard normal random numbers
      z = randn(n, length(mu));
  
      % Transform to multivariate normal
      y = L*z' + mu;
  
      y = y';
  end

  %    ___        _               _   
  %   / _ \ _   _| |_ _ __  _   _| |_ 
  %  | | | | | | | __| '_ \| | | | __|
  %  | |_| | |_| | |_| |_) | |_| | |_ 
  %   \___/ \__,_|\__| .__/ \__,_|\__|
  %                  |_|              
  function K_opt = compute_K_opt(model)
    % This function computes the local estimation of the global centroid, so where each agent thinks the network centroid is
    
      n_models = size(model, 1);
    
      K_opt = 0;
      for j=1:n_models
        K_opt = K_opt + model{j}.mu*model{j}.K_opt;
      end
      
     
  end

== matlab function winter_simulink_with_PC_generator_control_EKF/Torque reference/Torque_limit_part_load1/weighted_sum ==
  data: sigma_max input; y output; omega input; generator parameter
function y = fcn(sigma_max, omega, generator)

y = (1 - sigma_max)*generator.K_opt*omega^2 + ...
  sigma_max*generator.torque_full;

== matlab function winter_simulink_with_PC_generator_control_EKF/Torque reference/cubic_root1 ==
  data: u input; y output
function y = fcn(u)

y = nthroot(u, 3);

== matlab function winter_simulink_with_PC_generator_control_EKF/Torque reference/interpolation between limits1 ==
  data: Q_g_max output; Qg_part_min input; Qg_part_max input; Q_g_ref_full input; sigma_theta input; Q_g_min output
function [Q_g_max, Q_g_min] = fcn( Qg_part_min, ...
  Qg_part_max, Q_g_ref_full, sigma_theta)

Q_g_min = (1 - sigma_theta)*Qg_part_min + sigma_theta*Q_g_ref_full;
Q_g_max = (1 - sigma_theta)*Qg_part_max + sigma_theta*Q_g_ref_full;
